simulink model "MSE312ProjectGainSch2017b"  (R2018a)
settings: Solver=VariableStepAuto  StartTime=0.0  StopTime=10  RelTol=1e-3
libraries: simulink x2
settings Model: Creator=harri  LastModifiedBy=harri
settings CodeAppCC: StateflowObjectComments=on

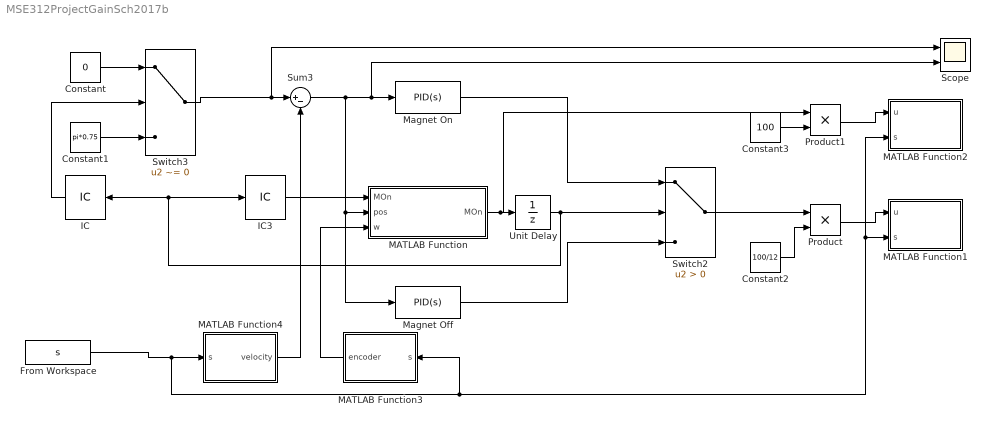
== system MSE312ProjectGainSch2017b ==
  Constant : Constant  Value=0
  Constant1 : Constant  Value=pi*0.75
  Constant2 : Constant  Value=100/12
  Constant3 : Constant  Value=100
  From Workspace : FromWorkspace  VariableName=s  SampleTime=0
  IC : InitialCondition  Value=0
  IC3 : InitialCondition  Value=0
  MATLAB Function : MATLAB Function  TreatAsAtomicUnit=on
  MATLAB Function1 : MATLAB Function  TreatAsAtomicUnit=on
  MATLAB Function2 : MATLAB Function  TreatAsAtomicUnit=on
  MATLAB Function3 : MATLAB Function  TreatAsAtomicUnit=on
  MATLAB Function4 : MATLAB Function  TreatAsAtomicUnit=on
  Magnet Off : simulink/Continuous/PID Controller  Controller=PID  Form=Parallel  TimeDomain=Continuous-time  SampleTime=-1  IntegratorMethod=Forward Euler  FilterMethod=Forward Euler  ControllerParametersSource=internal  P=10  I=0  D=2  UseFilter=on  N=100  TunerSelectOption=Transfer Function Based (PID Tuner App)  InitialConditionSource=internal  InitialConditionForIntegrator=0  InitialConditionForFilter=0  DifferentiatorICPrevScaledInput=0  ExternalReset=none  TrackingMode=off  Kt=1  LimitOutput=on  UpperSaturationLimit=12  LowerSaturationLimit=-12  LinearizeAsGain=on  AntiWindupMode=none  Kb=1  POutMin=[]  POutMax=[]  IOutMin=[]  IOutMax=[]  DOutMin=[]  DOutMax=[]  NOutMin=[]  NOutMax=[]  SumOutMin=[]  SumOutMax=[]  SaturationOutMin=[]  SaturationOutMax=[]  PParamMin=[]  PParamMax=[]  IParamMin=[]  IParamMax=[]  DParamMin=[]  DParamMax=[]  NParamMin=[]  NParamMax=[]  KbParamMin=[]  KbParamMax=[]  KtParamMin=[]  KtParamMax=[]  KbOutMin=[]  KbOutMax=[]  KtOutMin=[]  KtOutMax=[]  IntegratorOutMin=[]  IntegratorOutMax=[]  FilterOutMin=[]  FilterOutMax=[]  SumI1OutMin=[]  SumI1OutMax=[]  SumI2OutMin=[]  SumI2OutMax=[]  SumI3OutMin=[]  SumI3OutMax=[]  SumI4OutMin=[]  SumI4OutMax=[]  SumDOutMin=[]  SumDOutMax=[]  DifferentiatorOutMin=[]  DifferentiatorOutMax=[]  FilterDiffOutCoefMin=[]  FilterDiffOutCoefMax=[]  ReciprocalOutMin=[]  ReciprocalOutMax=[]  SumDenOutMin=[]  SumDenOutMax=[]  SumNumOutMin=[]  SumNumOutMax=[]  DivideOutMin=[]  DivideOutMax=[]  IntegratorContinuousStateAttributes=''  IntegratorStateMustResolveToSignalObject=off  IntegratorRTWStateStorageClass=Auto  FilterContinuousStateAttributes=''  FilterStateMustResolveToSignalObject=off  FilterRTWStateStorageClass=Auto  ParallelPVariant=InternalParameters  IdealPVariant=Disabled  IVariant=InternalParameters  DVariant=InternalParameters  IntegratorVariant=Continuous  SatVariant=Enabled  AWVariant=Passthrough  PCopyVariant=Disabled  TRVariant=Disabled  FdbkBlocksVariant=Forward  IdealPFdbkVariant=Disabled  SatFdbkVariant=Disabled  DerivativeFilterVariant=ContFilter  NVariant=InternalParameters  NCopyVariant=Disabled  FilterICVariant=InternalICsFilter  IntegratorICVariant=InternalICs  ExternalResetVariant=Disabled  TRSumVariant=Passthrough
  Magnet On : simulink/Continuous/PID Controller  Controller=PID  Form=Parallel  TimeDomain=Continuous-time  SampleTime=-1  IntegratorMethod=Forward Euler  FilterMethod=Forward Euler  ControllerParametersSource=internal  P=15  I=0  D=5  UseFilter=on  N=100  TunerSelectOption=Transfer Function Based (PID Tuner App)  InitialConditionSource=internal  InitialConditionForIntegrator=0  InitialConditionForFilter=0  DifferentiatorICPrevScaledInput=0  ExternalReset=none  TrackingMode=off  Kt=1  LimitOutput=on  UpperSaturationLimit=12  LowerSaturationLimit=-12  LinearizeAsGain=on  AntiWindupMode=none  Kb=1  POutMin=[]  POutMax=[]  IOutMin=[]  IOutMax=[]  DOutMin=[]  DOutMax=[]  NOutMin=[]  NOutMax=[]  SumOutMin=[]  SumOutMax=[]  SaturationOutMin=[]  SaturationOutMax=[]  PParamMin=[]  PParamMax=[]  IParamMin=[]  IParamMax=[]  DParamMin=[]  DParamMax=[]  NParamMin=[]  NParamMax=[]  KbParamMin=[]  KbParamMax=[]  KtParamMin=[]  KtParamMax=[]  KbOutMin=[]  KbOutMax=[]  KtOutMin=[]  KtOutMax=[]  IntegratorOutMin=[]  IntegratorOutMax=[]  FilterOutMin=[]  FilterOutMax=[]  SumI1OutMin=[]  SumI1OutMax=[]  SumI2OutMin=[]  SumI2OutMax=[]  SumI3OutMin=[]  SumI3OutMax=[]  SumI4OutMin=[]  SumI4OutMax=[]  SumDOutMin=[]  SumDOutMax=[]  DifferentiatorOutMin=[]  DifferentiatorOutMax=[]  FilterDiffOutCoefMin=[]  FilterDiffOutCoefMax=[]  ReciprocalOutMin=[]  ReciprocalOutMax=[]  SumDenOutMin=[]  SumDenOutMax=[]  SumNumOutMin=[]  SumNumOutMax=[]  DivideOutMin=[]  DivideOutMax=[]  IntegratorContinuousStateAttributes=''  IntegratorStateMustResolveToSignalObject=off  IntegratorRTWStateStorageClass=Auto  FilterContinuousStateAttributes=''  FilterStateMustResolveToSignalObject=off  FilterRTWStateStorageClass=Auto  ParallelPVariant=InternalParameters  IdealPVariant=Disabled  IVariant=InternalParameters  DVariant=InternalParameters  IntegratorVariant=Continuous  SatVariant=Enabled  AWVariant=Passthrough  PCopyVariant=Disabled  TRVariant=Disabled  FdbkBlocksVariant=Forward  IdealPFdbkVariant=Disabled  SatFdbkVariant=Disabled  DerivativeFilterVariant=ContFilter  NVariant=InternalParameters  NCopyVariant=Disabled  FilterICVariant=InternalICsFilter  IntegratorICVariant=InternalICs  ExternalResetVariant=Disabled  TRSumVariant=Passthrough
  Product : Product
  Product1 : Product
  Scope : Scope  NumInputPorts=2
  Sum3 : Sum  Inputs=|+-
  Switch2 : Switch  Criteria=u2 > Threshold
  Switch3 : Switch  Criteria=u2 ~= 0  Threshold=1  ZeroCross=off
  Unit Delay : UnitDelay  SampleTime=-1
  wires:
  Sum3/1 -> Magnet Off/1, MATLAB Function/2(pos), Scope/2, Magnet On/1
  Constant/1 -> Switch3/1
  Constant1/1 -> Switch3/3
  MATLAB Function4/1(velocity) -> Sum3/2
  MATLAB Function3/1(encoder) -> MATLAB Function/3(w)
  IC3/1 -> MATLAB Function/1("MOn ")
  MATLAB Function/1(MOn) -> Product1/1, Unit Delay/1
  Unit Delay/1 -> IC/1, IC3/1, Switch2/2
  Magnet Off/1 -> Switch2/3
  Magnet On/1 -> Switch2/1
  IC/1 -> Switch3/2
  Constant2/1 -> Product/2
  Constant3/1 -> Product1/2
  Switch2/1 -> Product/1
  Switch3/1 -> Scope/1, Sum3/1
  Product/1 -> MATLAB Function1/1(u)
  Product1/1 -> MATLAB Function2/1(u)
  From Workspace/1 -> MATLAB Function1/2(s), MATLAB Function2/2(s), MATLAB Function3/1(s), MATLAB Function4/1(s)

== matlab function MSE312ProjectGainSch2017b/MATLAB Function1 ==
  data: u input; s input
function PWM(u,s)

%Send speed (100)
fprintf(s,['s',num2str(u),13])

== matlab function MSE312ProjectGainSch2017b/MATLAB Function ==
  data: MOn input; MOn output; pos input; w input
function MOn  = GainSchedule(MOn, pos,w)

%%  Magnet On
if (MOn == 1) || ((abs(pos) < 0.1) && abs(w) < 0.1)
    MOn = 1;
end

== matlab function MSE312ProjectGainSch2017b/MATLAB Function2 ==
  data: u input; s input
function Magnet(u,s)

%Send magnet (100)
fprintf(s,['m',num2str(u),13])

== matlab function MSE312ProjectGainSch2017b/MATLAB Function3 ==
  data: encoder output; s input
function encoder = Position(s)
%get encoder
fprintf(s,['g',13])
encoder = str2num(fscanf(s))* (pi/6300);

== matlab function MSE312ProjectGainSch2017b/MATLAB Function4 ==
  data: velocity output; s input
function velocity = VelocityCOM(s)

%get velocity
fprintf(s,['v', 13]);
velocity = str2num(fscanf(s))/0.025 * (pi/6300);
